simulink model "ass2_2021b"  (R2021b)
settings: Solver=FixedStepAuto  StartTime=0.0  StopTime=inf  FixedStep=0.1  RelTol=1e-3
values from neighbouring files (symbols this model uses):
  wp1 = [5 0 pi/2]    [waypoints.m]
  wp10 = [0 0 3/2*pi]    [waypoints.m]
  wp2 = [5 5 5/4*pi]    [waypoints.m]
  wp3 = [-5 -5 pi/2]    [waypoints.m]
  wp4 = [-5 5 0]    [waypoints.m]
  wp5 = [0 0 0]    [waypoints.m]
  wp6 = [3 3 3/4*pi]    [waypoints.m]
  wp7 = [-3 0 3/2*pi]    [waypoints.m]
  wp8 = [0 -3 pi/4]    [waypoints.m]
  wp9 = [3 0 pi/2]    [waypoints.m]
undefined symbols (not defined in the file or in its folder): Angular, Linear
libraries: robotlib x5, simulink x1
settings Model: Creator=isa  LastModifiedBy=isabe
settings OptimizationCC: EnhancedBackFolding=on  PassReuseOutputArgsAs=Individual arguments  ZeroExternalMemoryAtStartup=off  ZeroInternalMemoryAtStartup=off  MaxStackSize=64  OptimizeBlockOrder=speed  DifferentSizesBufferReuse=on  OptimizationCustomize=off  EfficientTunableParamExpr=on
settings DebuggingCC: ParameterTunabilityLossMsg=error  UnconnectedInputMsg=none  UnconnectedOutputMsg=none  UnconnectedLineMsg=none
settings HardwareCC: ProdBitPerPointer=32  ProdBitPerSizeT=32  ProdBitPerPtrDiffT=32  ProdLargestAtomicFloat=None  ProdIntDivRoundTo=Undefined  ProdEndianess=Unspecified  ProdWordSize=32  ProdHWDeviceType=Generic->Unspecified (assume 32-bit Generic)
settings SFSimCC: MATLABDynamicMemAlloc=off
settings RTWCC: Description=Embedded Coder  SystemTargetFile=ert.tlc  HardwareBoard=Robot Operating System (ROS)  TLCOptions="-aInlineSetEventsForThisBaseRateFcn=TLC_FALSE -aSuppressMultiTaskScheduler=TLC_FALSE  -aRateBasedStepFcn=0"  TemplateMakefile=ert_default_tmf  Toolchain=Catkin  TargetLang=C++  DLArmComputeVersion=20.02.1
settings CodeAppCC: ForceParamTrailComments=on  IgnoreCustomStorageClasses=off  OperatorAnnotations=on  SimulinkDataObjDesc=on  SFDataObjDesc=on  InsertBlockDesc=on

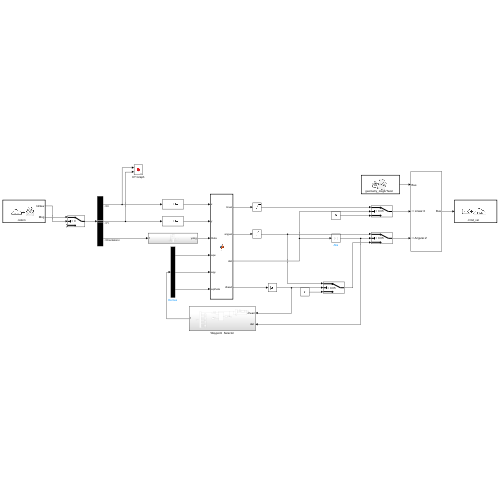
[thumbnail: Simulink's stored preview of the top-level diagram]
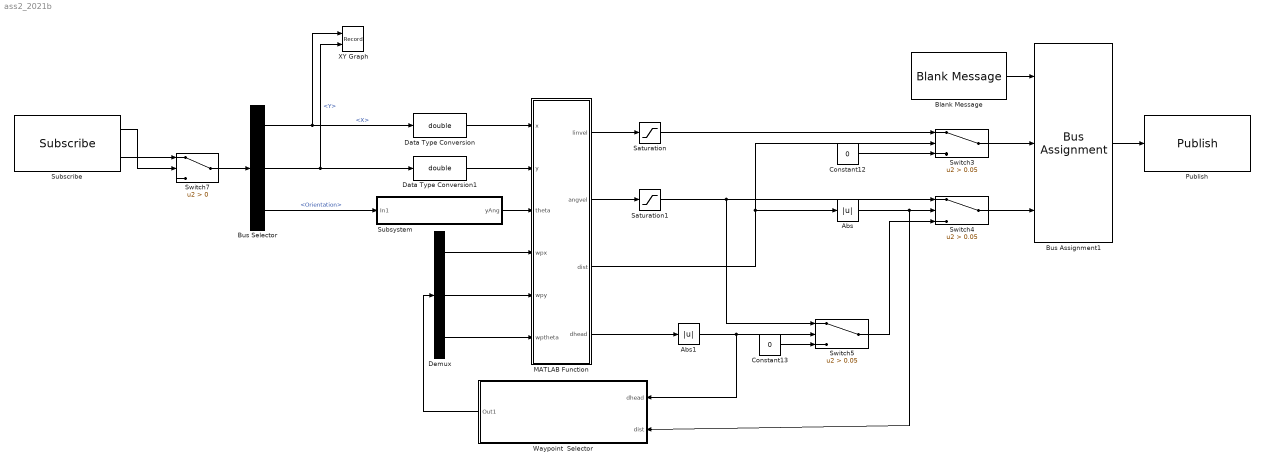
== system ass2_2021b ==
  Abs : Abs
  Abs1 : Abs
  Blank Message : robotlib/Blank Message  messageClass=Message  entityType=geometry_msgs/Twist  messageType=geometry_msgs/Twist  SampleTime=inf  legacyBusStruct=off
  Bus Assignment1 : BusAssignment  AssignedSignals=Linear.X,Angular.Z
  Bus Selector : BusSelector  OutputSignals=Pose.Pose.Position.X,Pose.Pose.Position.Y,Pose.Pose.Orientation
  Constant12 : Constant  Value=0
  Constant13 : Constant  Value=0
  Data Type Conversion : DataTypeConversion  OutDataTypeStr=double
  Data Type Conversion1 : DataTypeConversion  OutDataTypeStr=double
  Demux : Demux  Outputs=3
  MATLAB Function : MATLAB Function  TreatAsAtomicUnit=on
  Publish : robotlib/Publish  topicSource=Select from ROS network  topic=/cmd_vel  messageType=geometry_msgs/Twist  legacyBusStruct=off  messageQueueLength=1
  Saturation : Saturate  UpperLimit=0.2  LowerLimit=-0.2
  Saturation1 : Saturate  UpperLimit=0.4  LowerLimit=-0.4
  Subscribe : robotlib/Subscribe  topicSource=Specify your own  topic=/odom  messageType=nav_msgs/Odometry  SampleTime=-1  legacyBusStruct=off  messageQueueLength=1
  Subsystem : Subsystem
  Switch3 : Switch  Criteria=u2 > Threshold  Threshold=0.05
  Switch4 : Switch  Criteria=u2 > Threshold  Threshold=0.05
  Switch5 : Switch  Criteria=u2 > Threshold  Threshold=0.05
  Switch7 : Switch  Criteria=u2 > Threshold
  Waypoint  Selector : Subsystem
  XY Graph : Record  FileSettingsInternal="{\"entries\":[{\"content\":{\"excelSettings\":{\"content\":{},\"type\":\"Streamout.ExcelSettings\"}},\"type\":\"Streamout.FileSettingStorage\",\"uuid\":\"65f3e3c0-3afb-4dd5-a4a8-66a70b6ab4f2\"}],\"packageUris\":[\"http://schema.mathworks.com/mf0/streamout_blocks/R2020a\"],\"version\":\"1.0\"}"  Layout=[1 1]  SignalsInternal="{\"entries\":[{\"content\":{\"signals\":[{\"content\":{\"blockPath\":[\"ass2Prov_Switchcase2021b/XY Graph\"],\"channel\":[],\"dimensions\":[1],\"domain\":\"ass2Prov_Switchcase2021b/XY Graph\",\"lineColor\":\"#a2142f\",\"plots\":[1],\"port\":1,\"sid\":[],\"signalID\":9,\"signalName\":\"<X>\"},\"type\":\"RecordBlkView.Signal\",\"uuid\":\"1185a186-0d36-403c-a00f-c0733db3f458\"},{\"content\":{\"blockPath\":[\"ass2Prov_Switchcase2021b/XY Graph\"],\"channel\":[],\"dimensions\":[1],\"domain\":\"ass2Prov_Switchcase2021b/XY Graph\",\"lineColor\":\"#139fff\",\"plots\":[1],\"port\":2,\"sid\":[],\"signalID\":12,\"signalName\":\"<Y>\"},\"type\":\"RecordBlkView.Signal\",\"uuid\":\"add9b2c1-2869-48a2-be60-32ac011f313c\"}]},\"type\":\"RecordBlkView.InputSignals\",\"uuid\":\"6086c168-9bc6-49f6-b82c-43aa38b944a4\"}],\"packageUris\":[\"http://schema.mathworks.com/mf0/streamout_blocks/R2020a\"],\"version\":\"1.0\"}"  VisualizationBindings="{\"xyplotplugin\":{\"info\":[{\"series\":[{\"bindingParametersList\":[{\"parameter\":\"X-Axis\",\"signalID\":9,\"signalName\":\"<X>\"},{\"parameter\":\"Y-Axis\",\"signalID\":12,\"signalName\":\"<Y>\"}],\"seriesID\":45595}],\"subplotID\":1}]}}"  CompatibilityTag=XY  st=-1
  wires:
  Bus Assignment1/1 -> Publish/1
  Demux/1 -> MATLAB Function/4(wpx)
  Demux/2 -> MATLAB Function/5(wpy)
  Bus Selector/1 -> XY Graph/1, Data Type Conversion/1  "<X>"
  Bus Selector/2 -> XY Graph/2, Data Type Conversion1/1  "<Y>"
  MATLAB Function/1(linvel) -> Saturation/1
  MATLAB Function/2(angvel) -> Saturation1/1
  Data Type Conversion/1 -> MATLAB Function/1(x)
  Data Type Conversion1/1 -> MATLAB Function/2(y)
  Demux/3 -> MATLAB Function/6(wptheta)
  Bus Selector/3 -> Subsystem/1(In1)  "<Orientation>"
  Blank Message/1 -> Bus Assignment1/1
  Switch3/1 -> Bus Assignment1/2
  Switch4/1 -> Bus Assignment1/3
  Subsystem/1(yAng) -> MATLAB Function/3(theta)
  Subscribe/2 -> Switch7/1
  MATLAB Function/4(dhead) -> Abs1/1
  Saturation/1 -> Switch3/1
  Constant12/1 -> Switch3/3
  Constant13/1 -> Switch5/3
  Saturation1/1 -> Switch4/1, Switch5/1
  Switch5/1 -> Switch4/3
  MATLAB Function/3(dist) -> Switch3/2, Abs/1
  Subscribe/1 -> Switch7/2
  Switch7/1 -> Bus Selector/1
  Abs/1 -> Waypoint  Selector/2("dist "), Switch4/2
  Abs1/1 -> Switch5/2, Waypoint  Selector/1(dhead)
  Waypoint  Selector/1(Out1) -> Demux/1

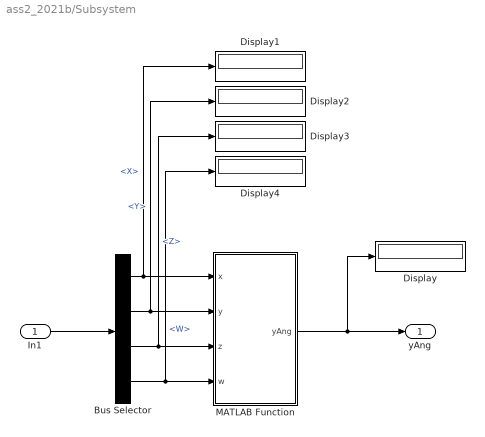
== system ass2_2021b/Subsystem ==
  In1 : Inport
  Bus Selector : BusSelector  OutputSignals=X,Y,Z,W
  Display{,1..4} (5 alike) : Display
  MATLAB Function : MATLAB Function  TreatAsAtomicUnit=on
  yAng : Outport
  wires:
  In1/1 -> Bus Selector/1
  MATLAB Function/1(yAng) -> Display/1, yAng/1
  Bus Selector/2 -> Display2/1, MATLAB Function/2(y)  "<Y>"
  Bus Selector/1 -> MATLAB Function/1(x), Display1/1  "<X>"
  Bus Selector/3 -> Display3/1, MATLAB Function/3(z)  "<Z>"
  Bus Selector/4 -> Display4/1, MATLAB Function/4(w)  "<W>"

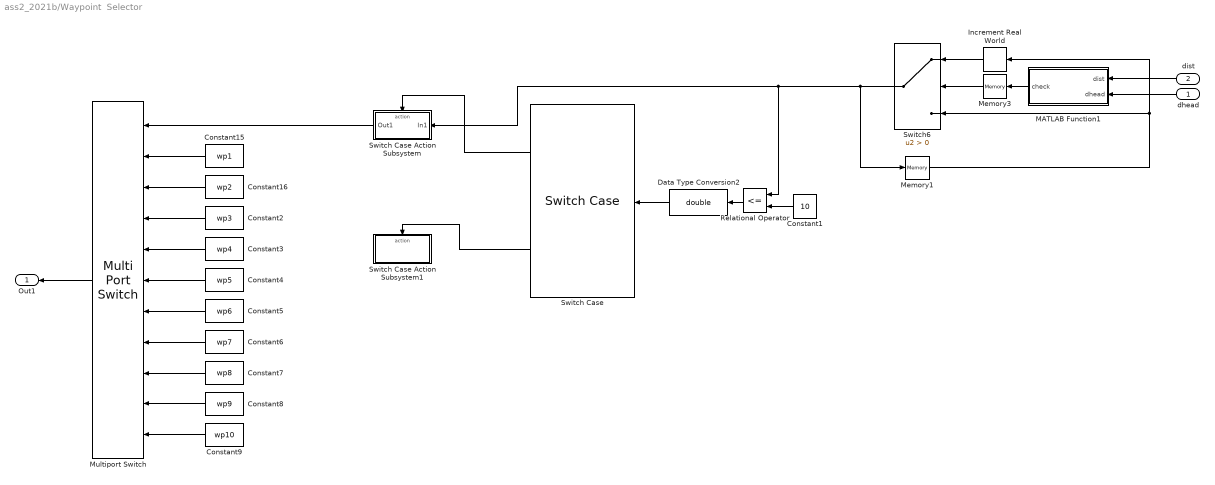
== system ass2_2021b/Waypoint  Selector ==
  dhead : Inport
  "dist " : Inport  Port=2
  Constant1 : Constant  Value=10
  Constant15 : Constant  Value=wp1
  Constant16 : Constant  Value=wp2
  Constant2 : Constant  Value=wp3
  Constant3 : Constant  Value=wp4
  Constant4 : Constant  Value=wp5
  Constant5 : Constant  Value=wp6
  Constant6 : Constant  Value=wp7
  Constant7 : Constant  Value=wp8
  Constant8 : Constant  Value=wp9
  Constant9 : Constant  Value=wp10
  Data Type Conversion2 : DataTypeConversion  OutDataTypeStr=double
  Increment Real World : simulink/Additional Math & Discrete/Additional Math: Increment - Decrement/Increment Real World
      settings: SourceProductBaseCode=SL
  MATLAB Function1 : MATLAB Function  TreatAsAtomicUnit=on
  Memory1 : Memory  InitialCondition=1
  Memory3 : Memory
  Multiport Switch : MultiPortSwitch  Inputs=10
  Relational Operator : RelationalOperator  Operator=<=  OutDataTypeStr=boolean  RndMeth=Simplest
  Switch Case : SwitchCase  CaseConditions={1,0}  ShowDefaultCase=off
  Switch Case Action Subsystem : Subsystem  TreatAsAtomicUnit=on
  Switch Case Action Subsystem1 : Subsystem  TreatAsAtomicUnit=on
  Switch6 : Switch  Criteria=u2 > Threshold
  Out1 : Outport
  wires:
  Constant5/1 -> Multiport Switch/7
  Constant7/1 -> Multiport Switch/9
  Constant3/1 -> Multiport Switch/5
  Constant4/1 -> Multiport Switch/6
  "dist "/1 -> MATLAB Function1/1(dist)
  Switch Case/2 -> Switch Case Action Subsystem1/Action
  Constant16/1 -> Multiport Switch/3
  Constant9/1 -> Multiport Switch/11
  MATLAB Function1/1(check) -> Memory3/1
  Multiport Switch/1 -> Out1/1
  Constant6/1 -> Multiport Switch/8
  Switch Case/1 -> Switch Case Action Subsystem/Action
  Constant1/1 -> Relational Operator/2
  Switch6/1 -> Memory1/1, Relational Operator/1, Switch Case Action Subsystem/1(In1)
  Constant8/1 -> Multiport Switch/10
  Relational Operator/1 -> Data Type Conversion2/1
  Switch Case Action Subsystem/1(Out1) -> Multiport Switch/1
  Constant2/1 -> Multiport Switch/4
  Constant15/1 -> Multiport Switch/2
  Data Type Conversion2/1 -> Switch Case/1
  Memory1/1 -> Increment Real World/1, Switch6/3
  Memory3/1 -> Switch6/2
  Increment Real World/1 -> Switch6/1
  dhead/1 -> MATLAB Function1/2(dhead)

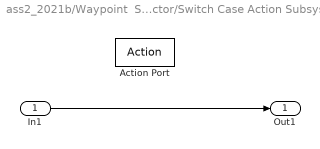
== system ass2_2021b/Waypoint  Selector/Switch Case Action Subsystem ==
  In1 : Inport
  Action Port : ActionPort  ActionPortLabel=case [ 1 ]:
  Out1 : Outport
  wires:
  In1/1 -> Out1/1

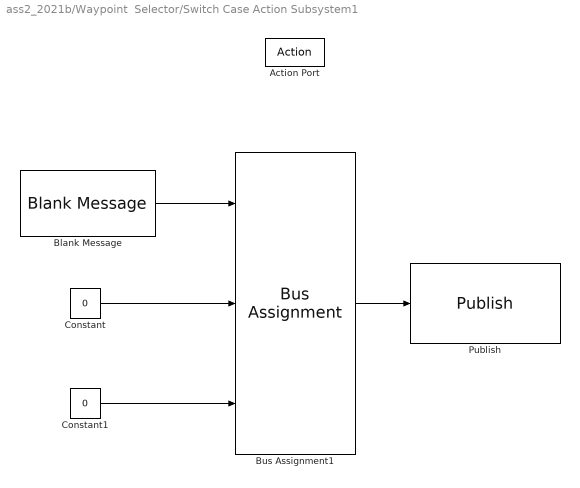
== system ass2_2021b/Waypoint  Selector/Switch Case Action Subsystem1 ==
  Action Port : ActionPort  ActionPortLabel=case [ 0 ]:
  Blank Message : robotlib/Blank Message  messageClass=Message  entityType=geometry_msgs/Twist  messageType=geometry_msgs/Twist  SampleTime=inf  legacyBusStruct=off
  Bus Assignment1 : BusAssignment  AssignedSignals=Linear.X,Angular.Z
  Constant : Constant  Value=0
  Constant1 : Constant  Value=0
  Publish : robotlib/Publish  topicSource=Select from ROS network  topic=/cmd_vel  messageType=geometry_msgs/Twist  legacyBusStruct=off  messageQueueLength=1
  wires:
  Blank Message/1 -> Bus Assignment1/1
  Constant/1 -> Bus Assignment1/2
  Bus Assignment1/1 -> Publish/1
  Constant1/1 -> Bus Assignment1/3

== matlab function ass2_2021b/Subsystem/MATLAB Function ==
  data: x input; yAng output; y input; z input; w input
function yAng = conversAngle(x,y,z,w)
eulAngle = quat2eul([w,x,y,z]);
yAng = eulAngle(1);
check = isnan(yAng);
if check == 1
    yAng = 0;
end
end

== matlab function ass2_2021b/MATLAB Function ==
  data: x input; linvel output; y input; theta input; wpx input; wpy input; angvel output; dist output; wptheta input; dhead output
function [linvel,angvel,dist,dhead] = fcn(x,y,theta,wpx,wpy,wptheta)
dist    = sqrt((x - wpx)^2 + (y - wpy)^2);
course  = atan2(wpy - y,wpx - x);

if dist <= 0.05 
    if theta < 0
        wptheta = wptheta - 2*pi;
    end
    dhead0 = 0;
    dhead = wptheta - theta;
else
    dhead0 = course - theta;
    if dhead0 < -pi
        dhead = dhead0 + 2*pi;
    elseif dhead0 > pi
        dhead = dhead0 - 2*pi;
    else
        dhead = dhead0;
    end
end

kpv     = 0.06;
kpw     = 0.05;
linvel  = kpv*dist;
angvel  = kpw*dhead;

end

== matlab function ass2_2021b/Waypoint  Selector/MATLAB Function1 ==
  data: dist input; check output; dhead input
function check = checkfc(dist,dhead)
if abs(dist) <= 0.05
    if abs(dhead) <= 0.05
        check = 1;
    else
        check = 0;
    end
else
    check = 0;
end
end
